simulink library "resettableRunningAverage"  (R2018a)
settings: Solver=VariableStepAuto  StartTime=0.0  StopTime=10.0  RelTol=1e-3
undefined symbols (not defined in the file): DiscIntNeverNeededParam
libraries: resettableTimer x1
settings Model: Creator=mitch  LastModifiedBy=mitch

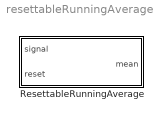
== system resettableRunningAverage ==
  ResettableRunningAverage : Subsystem

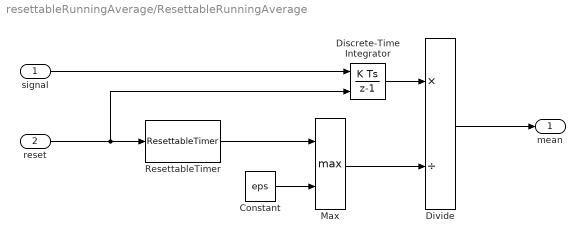
== system resettableRunningAverage/ResettableRunningAverage ==
  signal : Inport
  reset : Inport  Port=2
  Constant : Constant  Value=eps
  Discrete-Time Integrator : DiscreteIntegrator  ExternalReset=rising  SampleTime=-1  ICPrevOutput=DiscIntNeverNeededParam  ICPrevScaledInput=DiscIntNeverNeededParam
  Divide : Product  Inputs=*/
  Max : MinMax  Function=max  Inputs=2
  ResettableTimer : resettableTimer/ResettableTimer
  mean : Outport
  wires:
  Divide/1 -> mean/1
  Discrete-Time Integrator/1 -> Divide/1
  Max/1 -> Divide/2
  Constant/1 -> Max/2
  ResettableTimer/1 -> Max/1
  signal/1 -> Discrete-Time Integrator/1
  reset/1 -> ResettableTimer/1, Discrete-Time Integrator/2
